simulink model "ManualSimex"  (R2019a)
settings: Solver=FixedStepAuto  StartTime=0.0  StopTime=inf  RelTol=1e-3
undefined symbols (not defined in the file): gray
settings Model: EnablePacing=on  Creator=wuyua  LastModifiedBy=wuyua
settings DataIOCC: ReturnWorkspaceOutputs=off
settings DebuggingCC: ArithmeticOperatorsInVariantConditions=warning

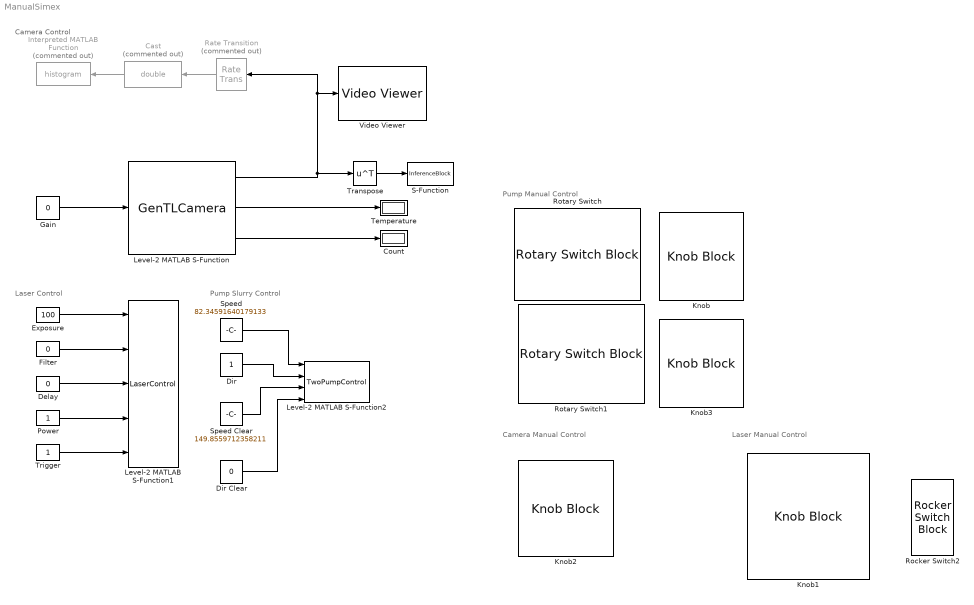
== system ManualSimex ==
  note: Camera Control
  note: Laser Control
  note: Pump Manual Control
  note: Pump Slurry Control
  note: Laser Manual Control
  note: Camera Manual Control
  Cast : DataTypeConversion  Commented=on  OutDataTypeStr=double
  Count : Display
  Delay : Constant  Value=0  OutDataTypeStr=uint32
  Dir : Constant  OutDataTypeStr=int8
  Dir Clear : Constant  Value=0  OutDataTypeStr=int8
  Exposure : Constant  Value=100  OutDataTypeStr=uint32
  Filter : Constant  Value=0  OutDataTypeStr=uint32
  Gain : Constant  Value=0
  Interpreted MATLAB Function : MATLABFcn  Commented=on  MATLABFcn=histogram  OutputDimensions=0
  Knob : KnobBlock  ScaleMax=500
  Knob1 : KnobBlock  ScaleMax=3000
  Knob2 : KnobBlock  ScaleMax=20
  Knob3 : KnobBlock  ScaleMax=500
  Level-2 MATLAB S-Function : M-S-Function  FunctionName=GenTLCamera
  Level-2 MATLAB S-Function1 : M-S-Function  FunctionName=LaserControl
  Level-2 MATLAB S-Function2 : M-S-Function  FunctionName=TwoPumpControl
  Power : Constant  OutDataTypeStr=uint8
  Rate Transition : RateTransition  Commented=on  OutPortSampleTime=1
  Rocker Switch2 : RockerSwitchBlock
      settings: Values={{'Off', 'On'}, [0 1]}
  Rotary Switch : RotarySwitchBlock
      settings: Values={{'Reverse', 'Stop', 'Forward'}, [-1 0 1]}
  Rotary Switch1 : RotarySwitchBlock
      settings: Values={{'Reverse', 'Stop', 'Forward'}, [-1 0 1]}
  S-Function : S-Function  FunctionName=InferenceBlock  Parameters=-1, 0  SFunctionDeploymentMode=off  EnableBusSupport=off
  Speed : Constant  Value=82.34591640179133  OutDataTypeStr=single
  Speed Clear : Constant  Value=149.8559712358211  OutDataTypeStr=single
  Temperature : Display
  Transpose : Math  Operator=transpose  SaturateOnIntegerOverflow=on
  Trigger : Constant  OutDataTypeStr=boolean
  Video Viewer : VideoViewer  colormapValue=gray(256)  FigPos=[287.4 824.4 766.4 716]
  wires:
  Level-2 MATLAB S-Function/2 -> Temperature/1
  Gain/1 -> Level-2 MATLAB S-Function/1
  Level-2 MATLAB S-Function/1 -> Transpose/1, Rate Transition/1, Video Viewer/1
  Filter/1 -> Level-2 MATLAB S-Function1/2
  Delay/1 -> Level-2 MATLAB S-Function1/3
  Power/1 -> Level-2 MATLAB S-Function1/4
  Trigger/1 -> Level-2 MATLAB S-Function1/5
  Speed/1 -> Level-2 MATLAB S-Function2/1
  Dir/1 -> Level-2 MATLAB S-Function2/2
  Dir Clear/1 -> Level-2 MATLAB S-Function2/4
  Speed Clear/1 -> Level-2 MATLAB S-Function2/3
  Level-2 MATLAB S-Function/3 -> Count/1
  Rate Transition/1 -> Cast/1
  Cast/1 -> Interpreted MATLAB Function/1
  Exposure/1 -> Level-2 MATLAB S-Function1/1
  Transpose/1 -> S-Function/1
